simulink model "derivace_funkce"  (R2021a)
settings: Solver=VariableStepAuto  StartTime=0.0  StopTime=10.0  RelTol=1e-3
libraries: simulink x1
settings Model: Creator=vojte  LastModifiedBy=vojte

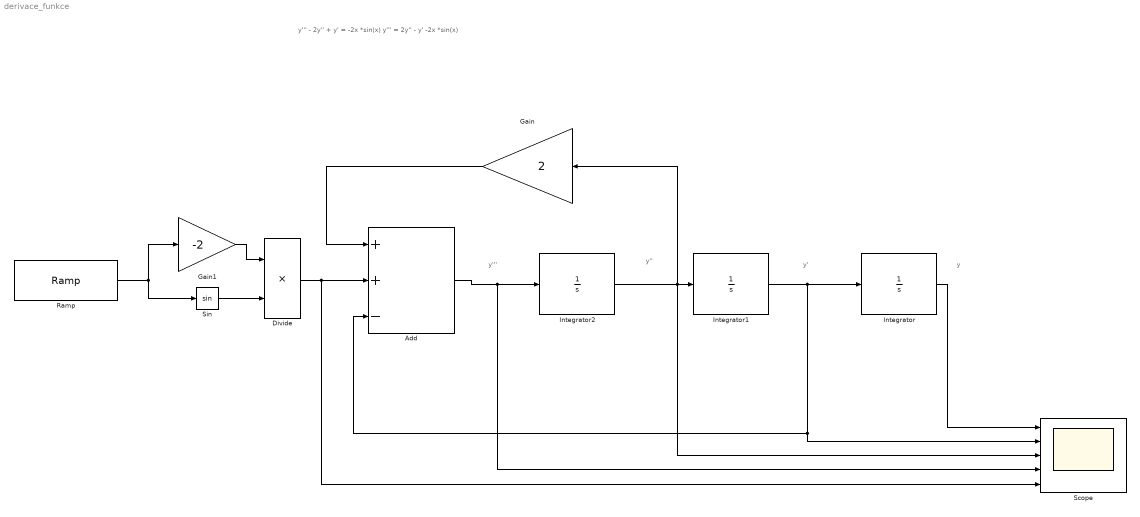
== system derivace_funkce ==
  note: y
  note: y'
  note: y''
  note: y'''
  note: y''' - 2y'' + y' = -2x *sin(x)
      | y''' = 2y'' - y' -2x *sin(x)
  Add : Sum  Inputs=++-
  Divide : Product  Inputs=**
  Gain : Gain  Gain=2
  Gain1 : Gain  Gain=-2
  Integrator : Integrator
  Integrator1 : Integrator
  Integrator2 : Integrator
  Ramp : simulink/Sources/Ramp  slope=1  start=0  InitialOutput=0
  Scope : Scope  NumInputPorts=5
  Sin : Trigonometry
  wires:
  Integrator/1 -> Scope/1
  Integrator1/1 -> Integrator/1, Scope/2, Add/3
  Integrator2/1 -> Scope/3, Gain/1, Integrator1/1
  Add/1 -> Scope/4, Integrator2/1
  Gain/1 -> Add/1
  Ramp/1 -> Sin/1, Gain1/1
  Gain1/1 -> Divide/1
  Sin/1 -> Divide/2
  Divide/1 -> Add/2, Scope/5
